simulink model "Junctions1False_tmp"  (Simulink 8.3)
settings: Solver=ode45  StartTime=0.0  StopTime=10.0  RelTol=1e-3
settings Model: Creator=scaife  LastModifiedBy=bourbouh  CovSFcnEnable=on  ExtModeAutoUpdateStatusClock=off
settings DataIOCC: SignalLoggingName=sigsOut
settings DebuggingCC: SaveWithParameterizedLinksMsg=none  SignalResolutionControl=TryResolveAllWithWarning  SolverPrmCheckMsg=none  MultiTaskDSMMsg=warning  MultiTaskCondExecSysMsg=none  FrameProcessingCompatibilityMsg=error  StateNameClashWarn=none
settings HardwareCC: TargetUnknown=on
settings SFSimCC: SimParseCustomCode=off

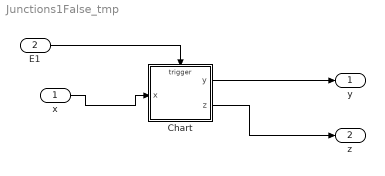
== system Junctions1False_tmp ==
  x : Inport
  E1 : Inport  Port=2
  Chart : Stateflow chart  TreatAsAtomicUnit=on
      settings: PermitHierarchicalResolution=ParametersOnly
  y : Outport
  z : Outport  Port=2
  wires:
  x/1 -> Chart/1(x)
  E1/1 -> Chart/Trigger
  Chart/1(y) -> y/1
  Chart/2(z) -> z/1

== stateflow chart Chart ==
  state A
    ex : y=y*2
  state C
  state B
  B -> A : [x>3]
  (default) -> A
  C -> A : [x>3]
  A -> (junction 10) [order 2] : [y>1]
  A -> (junction 11) [order 1] : E1[x>0]{y++}/z+=2
  (junction 11) -> C [order 3] : [x<2]{y++}/z++
  (junction 11) -> B [order 1] : [x>2]{y+=2}/z++
  (junction 10) -> C : [x==2]/z++
  (junction 11) -> (junction 12) [order 2] : [x==2]{y++}/z++
  (junction 12) -> C [order 2] : [y<=z]{y++}
  (junction 12) -> B [order 1] : [y>z]{y+=2}/z++
  data: x input int32; y output int32 =1; z output int32 =2
  events: E1 input EITHER_EDGE_EVENT
